simulink model "velocity_estimator_2016"  (R2016b)
settings: Solver=VariableStepAuto  StartTime=0.0  StopTime=10.0  RelTol=1e-3
libraries: marine_gnc x1
settings Model: Creator=mikkelsorensen  LastModifiedBy=mikkelsorensen

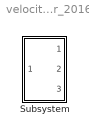
== system velocity_estimator_2016 ==
  Subsystem : Subsystem

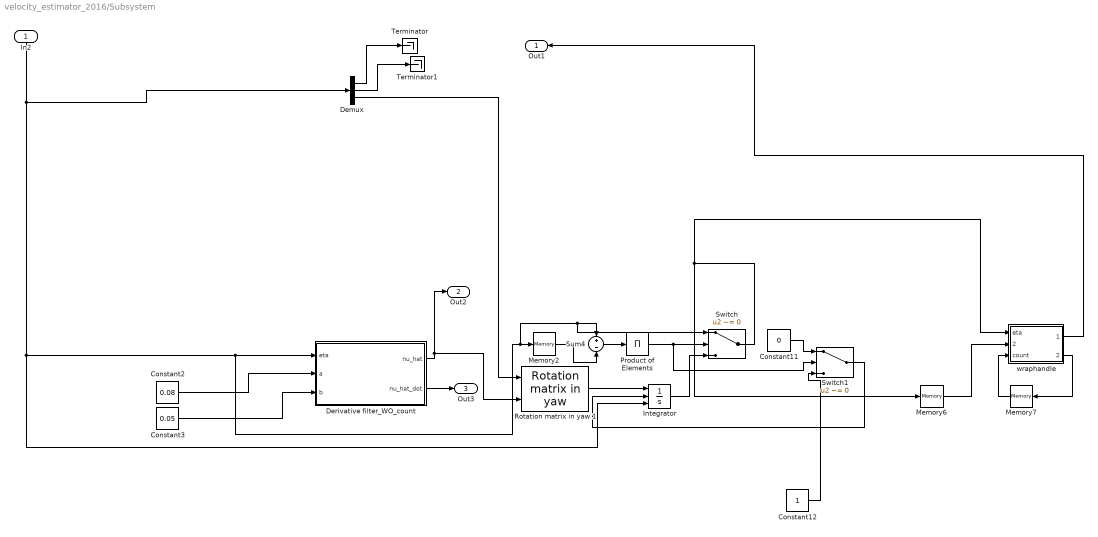
== system velocity_estimator_2016/Subsystem ==
  In2 : Inport
  Constant11 : Constant  Value=0
  Constant12 : Constant
  Constant2 : Constant  Value=0.08
  Constant3 : Constant  Value=0.05
  Demux : Demux  Outputs=3
  Derivative filter_WO_count : Subsystem
  Integrator : Integrator  ExternalReset=either  InitialConditionSource=external  InitialCondition=[0 0 0]
  Memory2 : Memory  X0=[0 0 0]
  Memory6 : Memory  X0=[0 0 0]
  Memory7 : Memory
  Product of Elements : Product  Inputs=*
  Rotation matrix in yaw 1 : marine_gnc/Models/ Kinematics/Rotation matrix in yaw 
  Sum4 : Sum  Inputs=+-
  Switch : Switch  Criteria=u2 ~= 0
  Switch1 : Switch  Criteria=u2 ~= 0
  Terminator : Terminator
  Terminator1 : Terminator
  wraphandle : MATLAB Function  TreatAsAtomicUnit=on
  Out1 : Outport
  Out2 : Outport  Port=2
  Out3 : Outport  Port=3
  wires:
  Constant2/1 -> Derivative filter_WO_count/2(a)
  Constant3/1 -> Derivative filter_WO_count/3(b)
  Derivative filter_WO_count/2(nu_hat_dot) -> Out3/1
  Rotation matrix in yaw 1/1 -> Integrator/1
  Memory2/1 -> Sum4/2
  wraphandle/1(eta_out) -> Out1/1
  Switch1/1 -> Integrator/2
  Integrator/1 -> Switch/3
  Constant11/1 -> Switch1/1
  Constant12/1 -> Switch1/3
  Sum4/1 -> Product of Elements/1
  Product of Elements/1 -> Switch1/2, Switch/2
  wraphandle/2(count_out) -> Memory7/1
  Memory7/1 -> wraphandle/3(count)
  Memory6/1 -> wraphandle/2(eta_prev)
  Switch/1 -> wraphandle/1(eta), Memory6/1
  Derivative filter_WO_count/1(nu_hat) -> Rotation matrix in yaw 1/2, Out2/1
  In2/1 -> Demux/1, Integrator/3, Switch/1, Sum4/1, Memory2/1, Derivative filter_WO_count/1(eta)
  Demux/3 -> Rotation matrix in yaw 1/1
  Demux/1 -> Terminator/1
  Demux/2 -> Terminator1/1

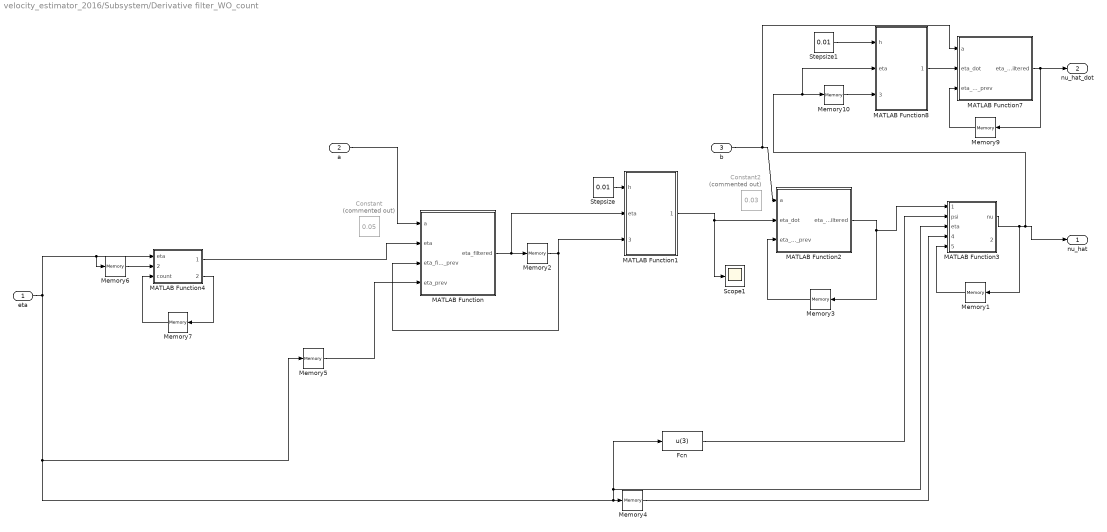
== system velocity_estimator_2016/Subsystem/Derivative filter_WO_count ==
  eta : Inport
  a : Inport  Port=2
  b : Inport  Port=3
  Constant : Constant  Commented=on  Value=0.05
  Constant2 : Constant  Commented=on  Value=0.03
  Fcn : Fcn  Expr=u(3)
  MATLAB Function : MATLAB Function  TreatAsAtomicUnit=on
  MATLAB Function1 : MATLAB Function  TreatAsAtomicUnit=on
  MATLAB Function2 : MATLAB Function  TreatAsAtomicUnit=on
  MATLAB Function3 : MATLAB Function  TreatAsAtomicUnit=on
  MATLAB Function4 : MATLAB Function  TreatAsAtomicUnit=on
  MATLAB Function7 : MATLAB Function  TreatAsAtomicUnit=on
  MATLAB Function8 : MATLAB Function  TreatAsAtomicUnit=on
  Memory{1..6,9..10} (8 alike) : Memory  X0=[0 0 0]
  Memory7 : Memory
  Scope1 : Scope
  Stepsize : Constant  Value=0.01
  Stepsize1 : Constant  Value=0.01
  nu_hat : Outport
  nu_hat_dot : Outport  Port=2
  wires:
  MATLAB Function7/1(eta_dot_filtered) -> Memory9/1, nu_hat_dot/1
  MATLAB Function4/2(count_out) -> Memory7/1
  Memory7/1 -> MATLAB Function4/3(count)
  Memory6/1 -> MATLAB Function4/2(eta_prev)
  MATLAB Function4/1(eta_out) -> MATLAB Function/2(eta)
  Stepsize1/1 -> MATLAB Function8/1(h)
  Memory10/1 -> MATLAB Function8/3(eta_prev)
  MATLAB Function8/1(eta_dot) -> MATLAB Function7/2(eta_dot)
  Memory9/1 -> MATLAB Function7/3(eta_dot_filtered_prev)
  eta/1 -> MATLAB Function4/1(eta), Memory6/1, Memory4/1, MATLAB Function3/3(eta), Fcn/1, Memory5/1
  Memory5/1 -> MATLAB Function/4(eta_prev)
  MATLAB Function3/1(nu) -> nu_hat/1, Memory10/1, MATLAB Function8/2(eta), Memory1/1
  Memory4/1 -> MATLAB Function3/4(prev_eta)
  Memory1/1 -> MATLAB Function3/5(prev_nu)
  MATLAB Function/1(eta_filtered) -> Memory2/1, MATLAB Function1/2(eta)
  b/1 -> MATLAB Function2/1(a), MATLAB Function7/1(a)
  a/1 -> MATLAB Function/1(a)
  Memory3/1 -> MATLAB Function2/3(eta_dot_filtered_prev)
  MATLAB Function2/1(eta_dot_filtered) -> Memory3/1, MATLAB Function3/1(eta_dot)
  MATLAB Function1/1(eta_dot) -> MATLAB Function2/2(eta_dot), Scope1/1
  Memory2/1 -> MATLAB Function/3(eta_filtered_prev), MATLAB Function1/3(eta_prev)
  Stepsize/1 -> MATLAB Function1/1(h)
  Fcn/1 -> MATLAB Function3/2(psi)

== matlab function velocity_estimator_2016/Subsystem/wraphandle ==
  data: eta input; eta_out output; eta_prev input; count input; count_out output
function [eta_out,count_out] = fcn(eta,eta_prev,count)

angle_d = eta(3)*180/pi;%+count*360;
angle = eta_prev(3)*180/pi;%+count*360;

angle_tilde = angle_d-angle;

if abs(angle_tilde)>300;
    count_out=-sign(angle_tilde)+count;
    angle_out=angle_d+count_out*360;
else
    count_out=count;
    angle_out=angle_d+count_out*360;
end

eta_out = eta;
eta_out(3) = angle_out*pi/180;


end

== matlab function velocity_estimator_2016/Subsystem/Derivative filter_WO_count/MATLAB Function ==
  data: a input; eta_filtered output; eta input; eta_filtered_prev input; eta_prev input
function eta_filtered  = fcn(a,eta,eta_filtered_prev,eta_prev)

psi = eta(3);
psitilde = psi-eta_prev(3);


eta_filtered = a*eta + (1-a)*eta_filtered_prev;

== matlab function velocity_estimator_2016/Subsystem/Derivative filter_WO_count/MATLAB Function1 ==
  data: h input; eta_dot output; eta input; eta_prev input
function eta_dot  = fcn(h,eta,eta_prev)

eta_tilde = eta-eta_prev;
eta_dot = (eta_tilde)./h;

if eta_dot(3)>5;
    eta_dot(3)=5;
elseif eta_dot(3)<-5;
   eta_dot(3)=-5; 
end

== matlab function velocity_estimator_2016/Subsystem/Derivative filter_WO_count/MATLAB Function2 ==
  data: a input; eta_dot_filtered output; eta_dot input; eta_dot_filtered_prev input
function eta_dot_filtered = fcn(a,eta_dot,eta_dot_filtered_prev)

eta_dot_filtered = a*eta_dot + (1-a)*eta_dot_filtered_prev;

== matlab function velocity_estimator_2016/Subsystem/Derivative filter_WO_count/MATLAB Function3 ==
  data: eta_dot input; nu output; psi input; eta input; prev_eta input; prev_nu input; count_out output
function [nu,count_out] = fcn(eta_dot,psi,eta,prev_eta,prev_nu)


if(prev_eta(1)==eta(1)||prev_eta(2)==eta(2)||prev_eta(3)==eta(3))
    nu = prev_nu;
    count_out =1;
else
    %if count == 1
        %nu = prev_nu;
        %count_out = 0;
    %else
        R_inv = [cos(psi)  sin(psi) 0
                 -sin(psi) cos(psi) 0
                 0         0        1];
        nu = R_inv*eta_dot;
        count_out = 0;
    %end
end

== matlab function velocity_estimator_2016/Subsystem/Derivative filter_WO_count/MATLAB Function4 ==
  data: eta input; eta_out output; eta_prev input; count input; count_out output
function [eta_out,count_out] = fcn(eta,eta_prev,count)

angle_d = eta(3)*180/pi;%+count*360;
angle = eta_prev(3)*180/pi;%+count*360;

angle_tilde = angle_d-angle;

if abs(angle_tilde)>300;
    count_out=-sign(angle_tilde)+count;
    angle_out=angle_d+count_out*360;
else
    count_out=count;
    angle_out=angle_d+count_out*360;
end

eta_out = eta;
eta_out(3) = angle_out*pi/180;


end

== matlab function velocity_estimator_2016/Subsystem/Derivative filter_WO_count/MATLAB Function7 ==
  data: a input; eta_dot_filtered output; eta_dot input; eta_dot_filtered_prev input
function eta_dot_filtered = fcn(a,eta_dot,eta_dot_filtered_prev)

eta_dot_filtered = a*eta_dot + (1-a)*eta_dot_filtered_prev;

== matlab function velocity_estimator_2016/Subsystem/Derivative filter_WO_count/MATLAB Function8 ==
  data: h input; eta_dot output; eta input; eta_prev input
function eta_dot  = fcn(h,eta,eta_prev)

eta_tilde = eta-eta_prev;
eta_dot = (eta_tilde)./h;

if eta_dot(3)>5;
    eta_dot(3)=5;
elseif eta_dot(3)<-5;
   eta_dot(3)=-5; 
end
